simulink model "Q1p7"  (R2018b)
settings: Solver=VariableStepAuto  StartTime=0.0  StopTime=10.0  RelTol=1e-3
values from neighbouring files (symbols this model uses):
  A = [0 1 0 0 0 0 ;  0 0 -10 0 -10 0; 0 0 0 1 0 0 ; 0 0 20 0 10 0 ; 0 0 0 0 0 1; 0 0 20 0 40 0]    [Q1part6.m]    (also in Q1part7.m; Q1part8.m; Q1part9.m)
  B = [0 1 0 -1 0 -2]'    [Q1part6.m]    (also in Q1part7.m; Q1part8.m; Q1part9.m)
  C = [0 0 1 0 0 0]    [Q1part6.m]    (also in Q1part7.m; Q1part8.m = [1 0 0 0 0 0; 0 0 1 0 0 0 ;0 0 0 0 1 0]; Q1part9.m = [1 0 0 0 0 0; 0 0 1 0 0 0 ;0 0 0 0 1 0])
  k = k3    [Q1part6.m]    (also in Q1part7.m = qi*alphaA; Q1part9.m = qi*alphaA)
settings Model: Creator=Asus  LastModifiedBy=Asus

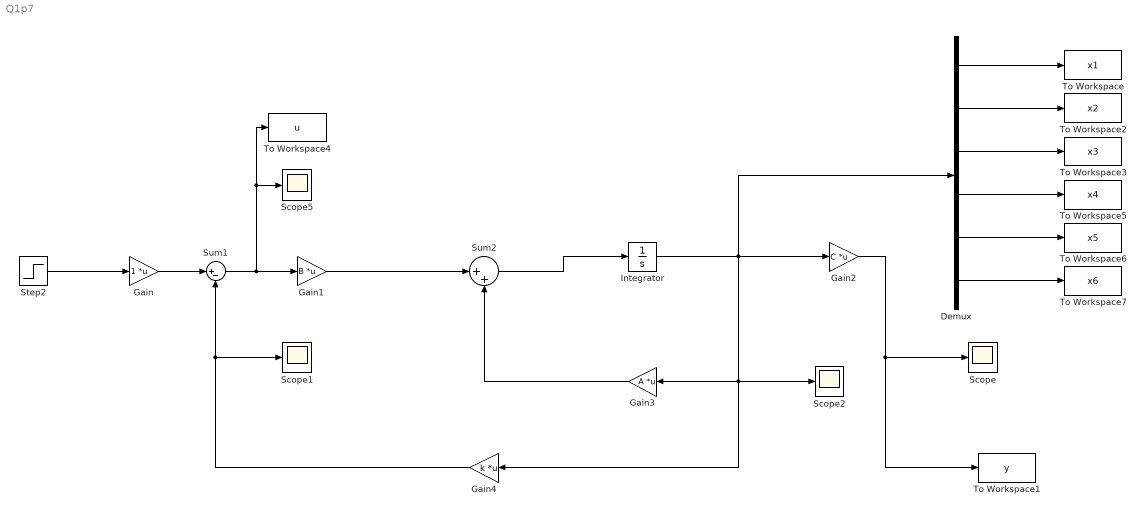
== system Q1p7 ==
  Demux : Demux  Outputs=6
  Gain : Gain  Multiplication=Matrix(K*u)
  Gain1 : Gain  Gain=B  Multiplication=Matrix(K*u)
  Gain2 : Gain  Gain=C  Multiplication=Matrix(K*u)
  Gain3 : Gain  Gain=A  Multiplication=Matrix(K*u)
  Gain4 : Gain  Gain=k  Multiplication=Matrix(K*u)
  Integrator : Integrator  InitialCondition=[0 0 0.1 0 -0.1 0]
  Scope{,1..2,5} (4 alike) : Scope
  Step2 : Step  Time=0  After=0  SampleTime=0
  Sum1 : Sum  Inputs=|+-
  Sum2 : Sum  Inputs=|++
  To Workspace : ToWorkspace  VariableName=x1  SaveFormat=Timeseries  SampleTime=-1
  To Workspace1 : ToWorkspace  VariableName=y  SaveFormat=Timeseries  SampleTime=-1
  To Workspace2 : ToWorkspace  VariableName=x2  SaveFormat=Timeseries  SampleTime=-1
  To Workspace3 : ToWorkspace  VariableName=x3  SaveFormat=Timeseries  SampleTime=-1
  To Workspace4 : ToWorkspace  VariableName=u  SaveFormat=Timeseries  SampleTime=-1
  To Workspace5 : ToWorkspace  VariableName=x4  SaveFormat=Timeseries  SampleTime=-1
  To Workspace6 : ToWorkspace  VariableName=x5  SaveFormat=Timeseries  SampleTime=-1
  To Workspace7 : ToWorkspace  VariableName=x6  SaveFormat=Timeseries  SampleTime=-1
  wires:
  Step2/1 -> Gain/1
  Gain3/1 -> Sum2/2
  Gain4/1 -> Scope1/1, Sum1/2
  Gain/1 -> Sum1/1
  Gain2/1 -> To Workspace1/1, Scope/1
  Integrator/1 -> Demux/1, Scope2/1, Gain4/1, Gain3/1, Gain2/1
  Gain1/1 -> Sum2/1
  Sum2/1 -> Integrator/1
  Demux/1 -> To Workspace/1
  Demux/2 -> To Workspace2/1
  Demux/3 -> To Workspace3/1
  Demux/4 -> To Workspace5/1
  Demux/5 -> To Workspace6/1
  Demux/6 -> To Workspace7/1
  Sum1/1 -> To Workspace4/1, Scope5/1, Gain1/1
